simulink model "ComparativoModeloReal"  (R2021a)
settings: Solver=VariableStepAuto  StartTime=0.0  StopTime=500  RelTol=1e-3
settings Model: Creator=Usuario  LastModifiedBy=Usuario

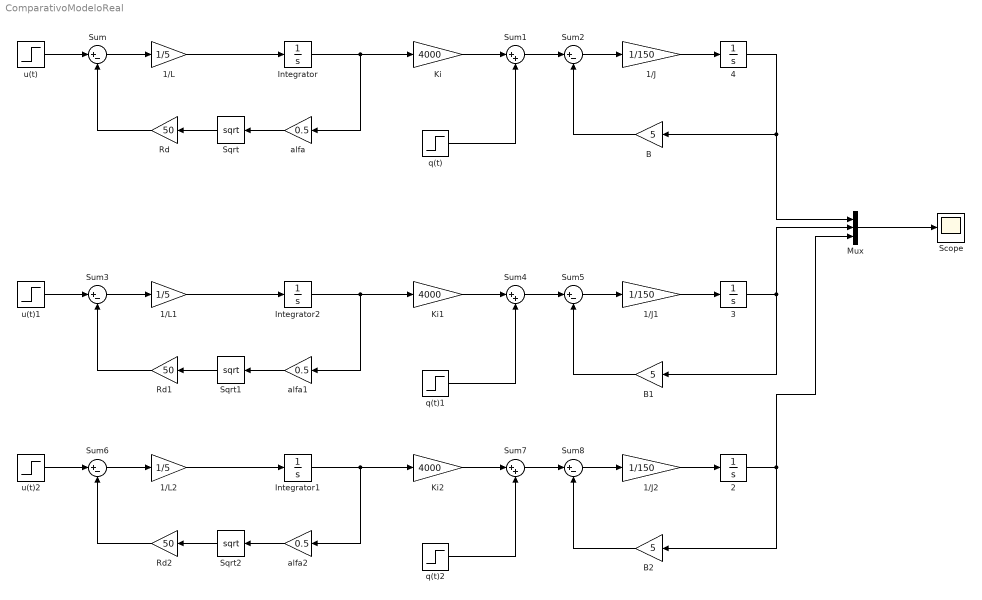
== system ComparativoModeloReal ==
  1/J : Gain  Gain=1/150
  1/J1 : Gain  Gain=1/150
  1/J2 : Gain  Gain=1/150
  1/L : Gain  Gain=1/5
  1/L1 : Gain  Gain=1/5
  1/L2 : Gain  Gain=1/5
  2 : Integrator
  3 : Integrator
  4 : Integrator
  B : Gain  Gain=5
  B1 : Gain  Gain=5
  B2 : Gain  Gain=5
  Integrator : Integrator
  Integrator1 : Integrator
  Integrator2 : Integrator
  Ki : Gain  Gain=4000
  Ki1 : Gain  Gain=4000
  Ki2 : Gain  Gain=4000
  Mux : Mux  Inputs=3
  Rd : Gain  Gain=50
  Rd1 : Gain  Gain=50
  Rd2 : Gain  Gain=50
  Scope : Scope
  Sqrt : Sqrt  SaturateOnIntegerOverflow=on
  Sqrt1 : Sqrt  SaturateOnIntegerOverflow=on
  Sqrt2 : Sqrt  SaturateOnIntegerOverflow=on
  Sum{,2..3,5..6,8} (6 alike) : Sum  Inputs=|+-
  Sum1 : Sum  Inputs=|++
  Sum4 : Sum  Inputs=|++
  Sum7 : Sum  Inputs=|++
  alfa : Gain  Gain=0.5
  alfa1 : Gain  Gain=0.5
  alfa2 : Gain  Gain=0.5
  q(t) : Step  Time=250  After=5  SampleTime=0
  q(t)1 : Step  Time=250  After=0  SampleTime=0
  q(t)2 : Step  Time=250  After=-5  SampleTime=0
  u(t) : Step  Time=250  Before=3  After=3  SampleTime=0
  u(t)1 : Step  Time=250  Before=3  After=3  SampleTime=0
  u(t)2 : Step  Time=250  Before=3  After=3  SampleTime=0
  wires:
  u(t)/1 -> Sum/1
  Sum/1 -> 1/L/1
  B/1 -> Sum2/2
  Sum2/1 -> 1/J/1
  1/L/1 -> Integrator/1
  Ki/1 -> Sum1/1
  q(t)/1 -> Sum1/2
  Integrator/1 -> alfa/1, Ki/1
  Sqrt/1 -> Rd/1
  Sum1/1 -> Sum2/1
  alfa/1 -> Sqrt/1
  1/J/1 -> 4/1
  4/1 -> Mux/1, B/1
  Rd/1 -> Sum/2
  u(t)1/1 -> Sum3/1
  Sum3/1 -> 1/L1/1
  B1/1 -> Sum5/2
  Sum5/1 -> 1/J1/1
  1/L1/1 -> Integrator2/1
  Ki1/1 -> Sum4/1
  q(t)1/1 -> Sum4/2
  Integrator2/1 -> alfa1/1, Ki1/1
  Sqrt1/1 -> Rd1/1
  Sum4/1 -> Sum5/1
  alfa1/1 -> Sqrt1/1
  1/J1/1 -> 3/1
  3/1 -> Mux/2, B1/1
  Rd1/1 -> Sum3/2
  u(t)2/1 -> Sum6/1
  Sum6/1 -> 1/L2/1
  B2/1 -> Sum8/2
  Sum8/1 -> 1/J2/1
  1/L2/1 -> Integrator1/1
  Ki2/1 -> Sum7/1
  q(t)2/1 -> Sum7/2
  Integrator1/1 -> alfa2/1, Ki2/1
  Sqrt2/1 -> Rd2/1
  Sum7/1 -> Sum8/1
  alfa2/1 -> Sqrt2/1
  1/J2/1 -> 2/1
  2/1 -> Mux/3, B2/1
  Rd2/1 -> Sum6/2
  Mux/1 -> Scope/1
